simulink model "VehCtrlMdel240926_2018b_amkspdlimit"  (R2019b)
settings: Solver=FixedStepDiscrete  StartTime=0.0  StopTime=30  FixedStep=0.0005  RelTol=1e-3  EnableMultiTasking=on
values from neighbouring files (symbols this model uses):
  Ldwf = 0.4    [VxSpdEstiPara.m]
  Ldwr = 0.5    [VxSpdEstiPara.m]
  thr1 = 0.5    [VxSpdEstiPara.m]
  thr2 = 0.5    [VxSpdEstiPara.m]
  thr3 = 0.5    [VxSpdEstiPara.m]
  thr4 = 0.5    [VxSpdEstiPara.m]
  TrqRquRate = 20    [VxSpdEstiPara.m]
undefined symbols (not defined in the file or in its folder): Ax_OffSet, Ay_OffSet, Caf, Car, DiscIntNeverNeededParam, dwf, dwr, h, i1, i2, I_AN02_28V, I_AN06_5V, I_AN07_5V, I_AN08_5V, I_AN09_5V, I_SW01_L, I_SW02_L, I_SW03_L, I_SW05_L, Iz, Kc, Ki, Kp, lf, lr, m, O_SW04_LS0A4, O_SW05_LS0A4, O_SW06_LS0A4, O_SW07_LS0A4, O_SW08_LS0A4, O_SW09_LS0A4, O_SW12_HS1A, O_SW13_HS1A, O_SW14_HS1A, O_SW15_HS1A, Offset_Angle, PWM3, Qa, Ra, RearRatio, Rt, thr5, YawRate_OffSet
libraries: simulink x158, ec5744lib x139, canmsglib x18, MyDesignedModel x1
(part 6 of 6)

== stateflow chart VehCtrlMdel240926_2018b_amkspdlimit/Drive_Ready/Subsystem/Chart2 ==
  state VehStat [parallel]
    settings: executionOrder=1
    state WaitForEngine
      en:
      send(AMKCANOFF,AMKCANenable);
      send(AMKDCOFF,AMKDCon);
      send(MCDCEnableOFF,MCDCEnable);
      send(InverterFLOFF,MCFL_InverterOn);
      send(InverterFROFF,MCFR_InverterOn);
      send(TorqueOFF,MC_TorqueCUT);
      errorReset = 0;
    state Standby
    state Trans
    state Guard
    state InitStateBack
    state Ready
    state Init
      en:
      errorReset = 1;
    state MCUReadyFail
    WaitForEngine -> Standby : [aMCUReady&&bMCUReady&&cMCUReady]
    Standby -> Guard [order 2] : [KeyPressed&&Brk&&ACC_Release&&cMCUReady&&aMCUReady&&bMCUReady&&aQuitInverterOn&&bQuitInverterOn]
    Trans -> Ready : after(2.5,sec){send(EbeepOFF,BeeperStat)}
    Guard -> Trans [order 1] : after(0.25,sec){send(EbeepON,BeeperStat)}
    Guard -> Standby [order 2] : [~KeyPressed||~Brk||~ACC_Release]
    Standby -> WaitForEngine [order 1] : [~aMCUReady||~bMCUReady||~cMCUReady]
    Guard -> InitStateBack [order 3] : [~cMCUReady||~aMCUReady||~bMCUReady]
    Init -> WaitForEngine : [after(0.1,sec)]
    MCUReadyFail -> WaitForEngine
    InitStateBack -> WaitForEngine
    (default) -> Init
    Ready -> MCUReadyFail : [~cMCUReady||~aMCUReady||~bMCUReady]
  state BeeperStat [parallel]
    settings: executionOrder=2
    state OFF
    state ON
    (default) -> BeeperStat.OFF
    BeeperStat.OFF -> BeeperStat.ON : EbeepON
    BeeperStat.ON -> BeeperStat.OFF : EbeepOFF
  state AMKDCon [parallel]
    settings: executionOrder=3
    state OFF
    state ON
    (default) -> AMKDCon.OFF
    AMKDCon.OFF -> AMKDCon.ON : AMKDCON
    AMKDCon.ON -> AMKDCon.OFF : AMKDCOFF
  state MCDCEnable [parallel]
    settings: executionOrder=4
    state OFF
    state ON
    (default) -> MCDCEnable.OFF
    MCDCEnable.OFF -> MCDCEnable.ON : MCDCEnableON
    MCDCEnable.ON -> MCDCEnable.OFF : MCDCEnableOFF
  state MC_TorqueCUT [parallel]
    settings: executionOrder=5
    state OFF
    state ON
    (default) -> MC_TorqueCUT.OFF
    MC_TorqueCUT.OFF -> MC_TorqueCUT.ON : TorqueON
    MC_TorqueCUT.ON -> MC_TorqueCUT.OFF : TorqueOFF
  state AMKDCready [parallel]
    settings: executionOrder=6
    state start
    state AMKCAN
      en:
      send(AMKCANON,AMKCANenable);
    state MC_DCready
    state MCDCOncheck
    state DCOnCheckPass
    state SYSRDYCECK
    state AMKDCOnFinish
      en:
      send(TorqueON,MC_TorqueCUT);
    state MCFR_InverterOn_State
      en:
      send(InverterFRON,MCFR_InverterOn);
    state MCFL_InverterOn_State
      en:
      send(InverterFLON,MCFL_InverterOn);
    state MCDCEnableState
      en:
      send(MCDCEnableON,MCDCEnable);
    (default) -> start
    MC_DCready -> MCDCOncheck : after(0.5,sec){send(AMKDCON,AMKDCon)}
    MCDCOncheck -> DCOnCheckPass : after(1,sec)
    AMKCAN -> MC_DCready : [KeyPressed&&Brk&&ACC_Release]
    start -> AMKCAN : after(5,sec)
    DCOnCheckPass -> MCDCEnableState : after(1,sec)[MCFLDCOncheck&&MCFRDCOncheck]
    SYSRDYCECK -> AMKDCOnFinish : after(8,sec)[MCFL_SYSREADY&&MCFR_SYSREADY&&aQuitInverterOn&&bQuitInverterOn]
    MCFR_InverterOn_State -> SYSRDYCECK : after(1,sec)
    MCFL_InverterOn_State -> MCFR_InverterOn_State : after(5,sec)
    MCDCEnableState -> MCFL_InverterOn_State : after(1,sec)
  state Output [parallel]
    du:
    VehReady = in(VehStat.Ready);
    VehStandby = in(VehStat.Standby);
    BeeperStOut = in(BeeperStat.ON);
    AMKCANready = in(AMKCANenable.ON);
    MCFL_DCOn_setpoints = in(AMKDCon.ON);
    MCFR_DCOn_setpoints = in(AMKDCon.ON);
    MCFL_DCEnable = in(MCDCEnable.ON);
    MCFR_DCEnable = in(MCDCEnable.ON);
    %MC_DCOnError = in(AMKDCready.MC_DCOnFail);
    AMKMCFL_InverterOn = in(MCFL_InverterOn.ON);
    AMKMCFR_InverterOn = in(MCFR_InverterOn.ON);
    MCFL_TorqueOn = in(MC_TorqueCUT.ON);
    MCFR_TorqueOn = in(MC_TorqueCUT.ON);
    settings: executionOrder=7
  state AMKCANenable [parallel]
    settings: executionOrder=8
    state OFF
    state ON
    (default) -> AMKCANenable.OFF
    AMKCANenable.OFF -> AMKCANenable.ON : AMKCANON
    AMKCANenable.ON -> AMKCANenable.OFF : AMKCANOFF
  state MCFL_InverterOn [parallel]
    settings: executionOrder=9
    state OFF
    state ON
    (default) -> MCFL_InverterOn.OFF
    MCFL_InverterOn.OFF -> MCFL_InverterOn.ON : InverterFLON
    MCFL_InverterOn.ON -> MCFL_InverterOn.OFF : InverterFLOFF
  state MCFR_InverterOn [parallel]
    settings: executionOrder=10
    state OFF
    state ON
    (default) -> MCFR_InverterOn.OFF
    MCFR_InverterOn.OFF -> MCFR_InverterOn.ON : InverterFRON
    MCFR_InverterOn.ON -> MCFR_InverterOn.OFF : InverterFROFF
  state MC_DCOnFail [parallel] [commented out]
    en:
    send(AMKDCOFF,AMKDCon);
    send(MCDCEnableOFF,MCDCEnable);
    send(InverterOFF,MC_InverterOn);
    send(TorqueOFF,MC_TorqueCUT);
  (default) -> MC_DCOnFail [commented out] : [~MCFRDCOncheck||~MCFLDCOncheck]
  (default) -> MC_DCOnFail [commented out] : [~MCFL_SYSREADY||~MCFR_SYSREADY||~aQuitInverterOn||~bQuitInverterOn]
  data: Brk input boolean size=1; KeyPressed input boolean size=1; VehReady output boolean size=1; BeeperStOut output boolean size=1; VehStandby output boolean; ACC_Release input boolean; cMCUReady input; aMCUReady input; bMCUReady input; AMKCANready output; MCFL_DCOn_setpoints output; MCFRDCOncheck input; MCFLDCOncheck input; MCFR_DCOn_setpoints output; MCFR_DCEnable output; MCFL_DCEnable output; MCFL_SYSREADY input; MCFR_SYSREADY input; errorReset output; aQuitInverterOn input; bQuitInverterOn input; MCFR_TorqueOn output; MCFL_TorqueOn output; AMKMCFL_InverterOn output; AMKMCFR_InverterOn output
  events: EbeepON local FUNCTION_CALL_EVENT; EbeepOFF local FUNCTION_CALL_EVENT; AMKCANOFF local FUNCTION_CALL_EVENT; AMKCANON local FUNCTION_CALL_EVENT; AMKDCON local FUNCTION_CALL_EVENT; AMKDCOFF local FUNCTION_CALL_EVENT; InverterOFF local FUNCTION_CALL_EVENT; InverterON local FUNCTION_CALL_EVENT; MCDCEnableON local FUNCTION_CALL_EVENT; MCDCEnableOFF local FUNCTION_CALL_EVENT; TorqueOFF local FUNCTION_CALL_EVENT; TorqueON local FUNCTION_CALL_EVENT; InverterFROFF local FUNCTION_CALL_EVENT; InverterFLOFF local FUNCTION_CALL_EVENT; InverterFLON local FUNCTION_CALL_EVENT; InverterFRON local FUNCTION_CALL_EVENT

== matlab function VehCtrlMdel240926_2018b_amkspdlimit/CTRL/MoTrqReq/DYC/MATLAB Function ==
  data: Fz1 input; T1max output; Fz2 input; Fz3 input; Fz4 input; T2max output; T34max output; TamkFL_max input; TamkFR_max input; Temrax_max input; ay_g input; Rt input; i1 input; i2 input; u input
function [T1max,T2max,T34max] = fcn(Fz1,Fz2,Fz3,Fz4, TamkFL_max,TamkFR_max, Temrax_max,ay_g,Rt,i1,i2,u)
g = 9.8;

Fx1 = sqrt(power(Fz1*u,2)-power(Fz1*ay_g/g,2));
Fx2 = sqrt(power(Fz2*u,2)-power(Fz2*ay_g/g,2));
Fx3 = sqrt(power(Fz3*u,2)-power(Fz3*ay_g/g,2));
Fx4 = sqrt(power(Fz4*u,2)-power(Fz4*ay_g/g,2));


T1max = min(Fx2*Rt/i1,TamkFR_max);
T2max = min(Fx1*Rt/i1,TamkFL_max);
T34max = min(min(Fx4,Fx3)*Rt/i2,Temrax_max);

== stateflow chart VehCtrlMdel240926_2018b_amkspdlimit/Input_Processing/Function-Call Subsystem/AccBrkPedal/Timer ==
  state Trigger
    en:
    x = x + 0.01;
    Exit=0;
  state Out
    en:
    Exit=1;
    x=0;
  state InterState
    en:
    x=0;
  Trigger -> Trigger [order 1] : [Trigger&&x<CountTime]
  Trigger -> Out [order 2] : [x>=CountTime]
  (default) -> Trigger
  Out -> Trigger : [~Trigger]
  InterState -> Trigger : [Trigger]
  Trigger -> InterState [order 3] : [x<CountTime&&~Trigger]
  data: Trigger input; CountTime input; Exit output; x local =0

== matlab function VehCtrlMdel240926_2018b_amkspdlimit/CTRL/MoTrqReq/DYC/MATLAB Function1 ==
  data: WSA input; Mz output; WSAV input; Vx input; Iz input; Caf input; Car input; lf input; lr input; m input
function Mz = fcn(WSA,WSAV,Vx,Iz,Caf,Car,lf,lr,m)

Mz = ((((lf*lf*Caf+lr*lr*Car)/Iz/Vx)*(-Caf/m/Vx)-((lf*Caf-lr*Car)/m/Vx/Vx-1)*(-lf*Caf/Iz))*Iz*WSA-(-Caf/m/Vx)*Iz*WSAV)/((lf*Caf-lr*Car)/m/Vx/Vx-1)/100;

== stateflow chart VehCtrlMdel240926_2018b_amkspdlimit/CTRL/PwrTrainTempPrtct/Timer1 ==
  state Trigger
    en:
    x = x + 0.01;
    Exit=0;
  state Out
    en:
    Exit=1;
    x=0;
  state InterState
    en:
    x=0;
  Trigger -> Trigger [order 1] : [Trigger&&x<CountTime]
  Trigger -> Out [order 2] : [x>=CountTime]
  (default) -> Trigger
  Out -> Trigger : [~Trigger]
  InterState -> Trigger : [Trigger]
  Trigger -> InterState [order 3] : [x<CountTime&&~Trigger]
  data: Trigger input; CountTime input; Exit output; x local =0

== stateflow chart VehCtrlMdel240926_2018b_amkspdlimit/CTRL/PwrTrainTempPrtct/Timer2 ==
  state Trigger
    en:
    x = x + 0.01;
    Exit=0;
  state Out
    en:
    Exit=1;
    x=0;
  state InterState
    en:
    x=0;
  Trigger -> Trigger [order 1] : [Trigger&&x<CountTime]
  Trigger -> Out [order 2] : [x>=CountTime]
  (default) -> Trigger
  Out -> Trigger : [~Trigger]
  InterState -> Trigger : [Trigger]
  Trigger -> InterState [order 3] : [x<CountTime&&~Trigger]
  data: Trigger input; CountTime input; Exit output; x local =0

== stateflow chart VehCtrlMdel240926_2018b_amkspdlimit/CTRL/MoTrqReq/Chart ==
  state A [parallel]
    settings: executionOrder=2
    state A
      en:
      if abs(IMU_Ay)>0.5
      a=atan(IMU_Ax/IMU_Ay)*180/pi;
      else
      a = 0;
      end
      b=sqrt(power(IMU_Ax,2)+power(IMU_Ay,2));
    (default) -> A.A
    A.A -> A.A
  state B [parallel]
    settings: executionOrder=1
    state InitState
    state DYC_Disenable
      en:
      DYC_Enable_OUT=0;
      DYC_flag=0;
    state DYC_Enable
      en:
      DYC_Enable_OUT=1;
      DYC_flag=1;
    (default) -> InitState
    DYC_Disenable -> InitState : [DYC_Enable]
    InitState -> DYC_Disenable [order 2] : [~DYC_Enable]
    DYC_Enable -> InitState : [IMU_Yaw>=50||IMU_Ay>=5||b>=5]
    InitState -> DYC_Enable [order 1] : [DYC_Enable&&IMU_Yaw<=50&&IMU_Ay<5&&b<5&&IMU_Yaw_Valid&&WhlStrAng_Valid]
  state C [parallel]
    settings: executionOrder=3
    state B
      en:
      TCSR_Enable_OUT=1;
    state F_TVD_TCS_STATE
    state C
      en:
      TCSR_Enable_OUT=0;
    F_TVD_TCS_STATE -> C.B [order 1] : [DYC_flag&&IMU_Yaw<=30&&a>=30&&a<=-30&&b<=3]
    C.B -> F_TVD_TCS_STATE : [~DYC_flag||IMU_Yaw>30||a>30||a>-30||b>3]
    (default) -> F_TVD_TCS_STATE
    C.C -> F_TVD_TCS_STATE : [DYC_flag&&IMU_Yaw<=30&&a>=30&&a<=-30&&b<=3]
    F_TVD_TCS_STATE -> C.C [order 2] : [~DYC_flag||IMU_Yaw>30||a>30||a>-30||b>3]
  state D [parallel]
    settings: executionOrder=4
    state InitState2
    state TCSR_Disenable
      en:
      TCSR_Enable_OUT=0;
    state TCSR_Enable
      en:
      TCSR_Enable_OUT=1;
    (default) -> InitState2
    InitState2 -> TCSR_Disenable [order 2] : [~TCSR_Enable]
    InitState2 -> TCSR_Enable [order 1] : [TCSR_Enable]
    TCSR_Disenable -> TCSR_Enable : [TCSR_Enable]
    TCSR_Enable -> TCSR_Disenable : [~TCSR_Enable]
  state E [parallel]
    settings: executionOrder=5
    state InitState1
    state TCSF_Disenable
      en:
      TCSF_Enable_OUT=0;
    state TCSF_Enable
      en:
      TCSF_Enable_OUT=1;
    (default) -> InitState1
    TCSF_Disenable -> InitState1 : [TCSF_Enable]
    InitState1 -> TCSF_Disenable [order 2] : [~TCSF_Enable]
    InitState1 -> TCSF_Enable [order 1] : [TCSF_Enable&&DYC_flag&&~DYC_flag&&a>60&&a<-60&&IMU_Ax>2&&b<5&&IMU_Yaw<50]
    TCSF_Enable -> InitState1 : [b>5]
  data: DYC_Enable input; TCSF_Enable input; TCSR_Enable input; TCSFR_flgActv input; TCSFL_flgActv input; TCSR_flgActv input; TVD_Trigger input; DYC_Enable_OUT output; TCSR_Enable_OUT output; TCSF_Enable_OUT output; IMU_Ax input; IMU_Ay input; IMU_Yaw input; a local; b local; DYC_flag local; IMU_Yaw_Valid input; WhlStrAng_Valid input

== stateflow chart VehCtrlMdel240926_2018b_amkspdlimit/Input_Processing/Function-Call Subsystem/SWAS/Timer ==
  state Trigger
    en:
    x = x + 0.01;
    Exit=0;
  state Out
    en:
    Exit=1;
    x=0;
  state InterState
    en:
    x=0;
  Trigger -> Trigger [order 1] : [Trigger&&x<CountTime]
  Trigger -> Out [order 2] : [x>=CountTime]
  (default) -> Trigger
  Out -> Trigger : [~Trigger]
  InterState -> Trigger : [Trigger]
  Trigger -> InterState [order 3] : [x<CountTime&&~Trigger]
  data: Trigger input; CountTime input; Exit output; x local =0

== stateflow chart VehCtrlMdel240926_2018b_amkspdlimit/Input_Processing/Function-Call Subsystem/WhlSpdii_mps/Timer ==
  state Trigger
    en:
    x = x + 0.01;
    Exit=0;
  state Out
    en:
    Exit=1;
    x=0;
  state InterState
    en:
    x=0;
  Trigger -> Trigger [order 1] : [Trigger&&x<CountTime]
  Trigger -> Out [order 2] : [x>=CountTime]
  (default) -> Trigger
  Out -> Trigger : [~Trigger]
  InterState -> Trigger : [Trigger]
  Trigger -> InterState [order 3] : [x<CountTime&&~Trigger]
  data: Trigger input; CountTime input; Exit output; x local =0

== stateflow chart VehCtrlMdel240926_2018b_amkspdlimit/Input_Processing/Function-Call Subsystem/WhlSpdii_mps/Timer1 ==
  state Trigger
    en:
    x = x + 0.01;
    Exit=0;
  state Out
    en:
    Exit=1;
    x=0;
  state InterState
    en:
    x=0;
  Trigger -> Trigger [order 1] : [Trigger&&x<CountTime]
  Trigger -> Out [order 2] : [x>=CountTime]
  (default) -> Trigger
  Out -> Trigger : [~Trigger]
  InterState -> Trigger : [Trigger]
  Trigger -> InterState [order 3] : [x<CountTime&&~Trigger]
  data: Trigger input; CountTime input; Exit output; x local =0

== stateflow chart VehCtrlMdel240926_2018b_amkspdlimit/Input_Processing/Function-Call Subsystem/WhlSpdii_mps/Timer2 ==
  state Trigger
    en:
    x = x + 0.01;
    Exit=0;
  state Out
    en:
    Exit=1;
    x=0;
  state InterState
    en:
    x=0;
  Trigger -> Trigger [order 1] : [Trigger&&x<CountTime]
  Trigger -> Out [order 2] : [x>=CountTime]
  (default) -> Trigger
  Out -> Trigger : [~Trigger]
  InterState -> Trigger : [Trigger]
  Trigger -> InterState [order 3] : [x<CountTime&&~Trigger]
  data: Trigger input; CountTime input; Exit output; x local =0

== stateflow chart VehCtrlMdel240926_2018b_amkspdlimit/Input_Processing/Function-Call Subsystem/WhlSpdii_mps/Timer3 ==
  state Trigger
    en:
    x = x + 0.01;
    Exit=0;
  state Out
    en:
    Exit=1;
    x=0;
  state InterState
    en:
    x=0;
  Trigger -> Trigger [order 1] : [Trigger&&x<CountTime]
  Trigger -> Out [order 2] : [x>=CountTime]
  (default) -> Trigger
  Out -> Trigger : [~Trigger]
  InterState -> Trigger : [Trigger]
  Trigger -> InterState [order 3] : [x<CountTime&&~Trigger]
  data: Trigger input; CountTime input; Exit output; x local =0

== matlab function VehCtrlMdel240926_2018b_amkspdlimit/CTRL/MoTrqReq/DYC/Wtarget ==
  data: Vx_mps input size=1; Wtarget output size=1; WhlStrAng input size=1; btarget output; lf input; lr input; m input; Car input; Caf input; u input; Ax_mpss input
function [Wtarget,btarget] = fcn(Vx_mps,WhlStrAng,lf,lr,m,Car,Caf,u,Ax_mpss)
Wdes = Vx_mps*WhlStrAng/(lf+lr+(m*Vx_mps*Vx_mps*(lr*Car-lf*Caf)/Caf/Car/(lr+lf)/2));
Wu = 0.8*u*9.8/Ax_mpss;
temp = min(abs(Wu),abs(Wdes));
    Wtarget = 0.8*temp*sign(Wdes);
%     Wtarget = Wdes;

bdes = (lr-lf*m*Vx_mps*Vx_mps/Car/(lf+lr)/2)*WhlStrAng/(lr+lf+m*Vx_mps*Vx_mps*(lr*Car-lf*Caf)/Car/Caf/(lf+lr)/2);
bu = atan(0.02*u*9.8);
if abs(bdes)<=bu
btarget = bdes;
else
    btarget = bu*sign(bdes);
end

== stateflow chart VehCtrlMdel240926_2018b_amkspdlimit/Input_Processing/Subsystem/WhlSlpageJudgment/Timer ==
  state Trigger
    en:
    x = x + 0.01;
    Exit=0;
  state Out
    en:
    Exit=1;
    x=0;
  state InterState
    en:
    x=0;
  Trigger -> Trigger [order 1] : [Trigger&&x<CountTime]
  Trigger -> Out [order 2] : [x>=CountTime]
  (default) -> Trigger
  Out -> Trigger : [~Trigger]
  InterState -> Trigger : [Trigger]
  Trigger -> InterState [order 3] : [x<CountTime&&~Trigger]
  data: Trigger input; CountTime input; Exit output; x local =0

== stateflow chart VehCtrlMdel240926_2018b_amkspdlimit/Input_Processing/Subsystem/WhlSpdSelect/Timer1 ==
  state Trigger
    en:
    x = x + 0.01;
    Exit=0;
  state Out
    en:
    Exit=1;
    x=0;
  state InterState
    en:
    x=0;
  Trigger -> Trigger [order 1] : [Trigger&&x<CountTime]
  Trigger -> Out [order 2] : [x>=CountTime]
  (default) -> Trigger
  Out -> Trigger : [~Trigger]
  InterState -> Trigger : [Trigger]
  Trigger -> InterState [order 3] : [x<CountTime&&~Trigger]
  data: Trigger input; CountTime input; Exit output; x local =0

== stateflow chart VehCtrlMdel240926_2018b_amkspdlimit/Input_Processing/Subsystem/WhlSpdSelect/Timer2 ==
  state Trigger
    en:
    x = x + 0.01;
    Exit=0;
  state Out
    en:
    Exit=1;
    x=0;
  state InterState
    en:
    x=0;
  Trigger -> Trigger [order 1] : [Trigger&&x<CountTime]
  Trigger -> Out [order 2] : [x>=CountTime]
  (default) -> Trigger
  Out -> Trigger : [~Trigger]
  InterState -> Trigger : [Trigger]
  Trigger -> InterState [order 3] : [x<CountTime&&~Trigger]
  data: Trigger input; CountTime input; Exit output; x local =0

== stateflow chart VehCtrlMdel240926_2018b_amkspdlimit/Input_Processing/Subsystem/WhlSlpageJudgment/Timer1 ==
  state Trigger
    en:
    x = x + 0.01;
    Exit=0;
  state Out
    en:
    Exit=1;
    x=0;
  state InterState
    en:
    x=0;
  Trigger -> Trigger [order 1] : [Trigger&&x<CountTime]
  Trigger -> Out [order 2] : [x>=CountTime]
  (default) -> Trigger
  Out -> Trigger : [~Trigger]
  InterState -> Trigger : [Trigger]
  Trigger -> InterState [order 3] : [x<CountTime&&~Trigger]
  data: Trigger input; CountTime input; Exit output; x local =0

== stateflow chart VehCtrlMdel240926_2018b_amkspdlimit/Input_Processing/Subsystem/WhlSlpageJudgment/Timer2 ==
  state Trigger
    en:
    x = x + 0.01;
    Exit=0;
  state Out
    en:
    Exit=1;
    x=0;
  state InterState
    en:
    x=0;
  Trigger -> Trigger [order 1] : [Trigger&&x<CountTime]
  Trigger -> Out [order 2] : [x>=CountTime]
  (default) -> Trigger
  Out -> Trigger : [~Trigger]
  InterState -> Trigger : [Trigger]
  Trigger -> InterState [order 3] : [x<CountTime&&~Trigger]
  data: Trigger input; CountTime input; Exit output; x local =0

== stateflow chart VehCtrlMdel240926_2018b_amkspdlimit/Input_Processing/Subsystem/WhlSlpageJudgment/Timer3 ==
  state Trigger
    en:
    x = x + 0.01;
    Exit=0;
  state Out
    en:
    Exit=1;
    x=0;
  state InterState
    en:
    x=0;
  Trigger -> Trigger [order 1] : [Trigger&&x<CountTime]
  Trigger -> Out [order 2] : [x>=CountTime]
  (default) -> Trigger
  Out -> Trigger : [~Trigger]
  InterState -> Trigger : [Trigger]
  Trigger -> InterState [order 3] : [x<CountTime&&~Trigger]
  data: Trigger input; CountTime input; Exit output; x local =0

== matlab function VehCtrlMdel240926_2018b_amkspdlimit/CTRL/MoTrqReq/DYC/载荷转移 ==
  data: ax input; Fz1 output; Fz2 output; Fz3 output; Fz4 output; ay input; h input; lfw input; lrw input; lf input; lr input; m input
function [Fz1,Fz2,Fz3,Fz4] = fcn(ax,ay,h,lfw,lrw,lf,lr,m)
g = 9.8;

Fz1 = (lr/(lf+lr))*(0.5*m*g-m*ay*h/lfw)-0.5*m*ax*h/(lf+lr);
Fz2 = (lr/(lf+lr))*(0.5*m*g+m*ay*h/lfw)-0.5*m*ax*h/(lf+lr);
Fz3 = (lr/(lf+lr))*(0.5*m*g-m*ay*h/lrw)+0.5*m*ax*h/(lf+lr);
Fz4 = (lr/(lf+lr))*(0.5*m*g+m*ay*h/lrw)+0.5*m*ax*h/(lf+lr);

== stateflow chart VehCtrlMdel240926_2018b_amkspdlimit/Input/key/Timer ==
  state Trigger
    en:
    x = x + 0.01;
    Exit=0;
  state Out
    en:
    Exit=1;
    x=0;
  state InterState
    en:
    x=0;
  Trigger -> Trigger [order 1] : [Trigger&&x<CountTime]
  Trigger -> Out [order 2] : [x>=CountTime]
  (default) -> Trigger
  Out -> Trigger : [~Trigger]
  InterState -> Trigger : [Trigger]
  Trigger -> InterState [order 3] : [x<CountTime&&~Trigger]
  data: Trigger input; CountTime input; Exit output; x local =0

== stateflow chart VehCtrlMdel240926_2018b_amkspdlimit/OUTPUT/Beeper/Timer1 ==
  state Trigger
    en:
    x = x + 0.01;
    Exit=1;
  state Out
    en:
    Exit=0;
    x=0;
  state InterState
    en:
    x=0;
  Trigger -> Trigger [order 1] : [~Trigger&&x<CountTime]
  Trigger -> Out [order 2] : [x>=CountTime]
  (default) -> Trigger
  Out -> Trigger : [Trigger]
  InterState -> Trigger : [~Trigger]
  Trigger -> InterState [order 3] : [x<CountTime&&Trigger]
  data: Trigger input; CountTime input; Exit output; x local =0

== stateflow chart VehCtrlMdel240926_2018b_amkspdlimit/Input/key/Timer1 ==
  state Trigger
    en:
    x = x + 0.01;
    Exit=0;
  state Out
    en:
    Exit=1;
    x=0;
  state InterState
    en:
    x=0;
  Trigger -> Trigger [order 1] : [~Trigger&&x<CountTime]
  Trigger -> Out [order 2] : [x>=CountTime]
  (default) -> Trigger
  Out -> Trigger : [Trigger]
  InterState -> Trigger : [~Trigger]
  Trigger -> InterState [order 3] : [x<CountTime&&Trigger]
  data: Trigger input; CountTime input; Exit output; x local =0

== stateflow chart VehCtrlMdel240926_2018b_amkspdlimit/OUTPUT/Beeper/Chart ==
  state STATEON
    state initstate
      en:
      VCUEnable=false;
    state ON
      en:
      VCUEnable=true;
    (default) -> initstate
    initstate -> ON : after(0.2,sec)[out1]
  state STATEOFF
    state initstate1
      en:
      VCUEnable=true;
    state OFF
      en:
      VCUEnable=false;
    (default) -> initstate1
    initstate1 -> OFF : after(0.2,sec)[out1]
  (default) -> STATEON
  ON -> STATEOFF
  OFF -> STATEON
  data: out1 input boolean; VCUEnable output boolean

== stateflow chart VehCtrlMdel240926_2018b_amkspdlimit/OUTPUT/Beeper/Timer2 ==
  state Trigger
    en:
    x = x + 0.01;
    Exit=0;
  state Out
    en:
    Exit=1;
    x=0;
  state InterState
    en:
    x=0;
  Trigger -> Trigger [order 1] : [Trigger&&x<CountTime]
  Trigger -> Out [order 2] : [x>=CountTime]
  (default) -> Trigger
  Out -> Trigger : [~Trigger]
  InterState -> Trigger : [Trigger]
  Trigger -> InterState [order 3] : [x<CountTime&&~Trigger]
  data: Trigger input; CountTime input; Exit output; x local =0

== matlab function VehCtrlMdel240926_2018b_amkspdlimit/CTRL/MoTrqReq/Subsystem/Subsystem/MATLAB Function ==
  data: u input; R1 output; R2 output; R3 output
function [R1,R2,R3] = fcn(u)

y1 = u(1,1);
y2 = u(2,2);
y3 = u(3,3);
R1 = y1/(y1+y2+y3);
R2 = y2/(y1+y2+y3);
R3 = y3/(y1+y2+y3);

== stateflow chart VehCtrlMdel240926_2018b_amkspdlimit/OUTPUT/Beeper/Enabled Subsystem1/Chart ==
  state Init
  state StateA
    state LEDON
      en:
      LEDOn=0;
    state LEDOFF
      en:
      LEDOn=1;
    StateA.LEDON -> StateA.LEDOFF : after(0.8,sec)
    (default) -> StateA.LEDON
    StateA.LEDOFF -> StateA.LEDON : after(0.8,sec)
  state StateB
    state LEDON
      en:
      LEDOn=0;
    state LEDOFF
      en:
      LEDOn=1;
    StateB.LEDON -> StateB.LEDOFF : after(0.4,sec)
    (default) -> StateB.LEDON
    StateB.LEDOFF -> StateB.LEDON : after(0.4,sec)
  state StateC
    state LEDON
      en:
      LEDOn=0;
    state LEDOFF
      en:
      LEDOn=1;
    StateC.LEDON -> StateC.LEDOFF : after(0.1,sec)
    (default) -> StateC.LEDON
    StateC.LEDOFF -> StateC.LEDON : after(0.1,sec)
  (default) -> Init
  Init -> StateA [order 1] : [FL&&~FR]
  StateA -> Init : [~FL||FR]
  Init -> StateB [order 2] : [~FL&&FR]
  StateB -> Init : [FL||~FR]
  Init -> StateC [order 3] : [FL&&FR]
  StateC -> Init : [~FL||~FR]
  data: LEDOn output; FR input; FL input

== stateflow chart VehCtrlMdel240926_2018b_amkspdlimit/Input_Processing/Function-Call Subsystem/Subsystem1/Chart ==
  state STATEON
    state initstate
      en:
      Trq_CUT=false;
    state ON
      en:
      Trq_CUT=true;
    (default) -> initstate
    initstate -> ON : after(0.2,sec)[out1]
  state STATEOFF
    state initstate1
      en:
      Trq_CUT=true;
    (default) -> initstate1
  (default) -> STATEON
  ON -> STATEOFF
  data: out1 input boolean; Trq_CUT output

== stateflow chart VehCtrlMdel240926_2018b_amkspdlimit/Input_Processing/Function-Call Subsystem/Subsystem1/Timer ==
  state Trigger
    en:
    x = x + 0.01;
    Exit=0;
  state Out
    en:
    Exit=1;
    x=0;
  state InterState
    en:
    x=0;
  Trigger -> Trigger [order 1] : [Trigger&&x<CountTime]
  Trigger -> Out [order 2] : [x>=CountTime]
  (default) -> Trigger
  Out -> Trigger : [~Trigger]
  InterState -> Trigger : [Trigger]
  Trigger -> InterState [order 3] : [x<CountTime&&~Trigger]
  data: Trigger input; CountTime input; Exit output; x local =0
